simulink model "ex3bSim"  (R2023b)
settings: Solver=VariableStepAuto  StartTime=0.0  StopTime=1000  RelTol=1e-3
values from neighbouring files (symbols this model uses):
  ki = 2    [ex3b.m]
  kp = 2    [ex3b.m]
settings Model: Creator=Bianca  LastModifiedBy=Bianca

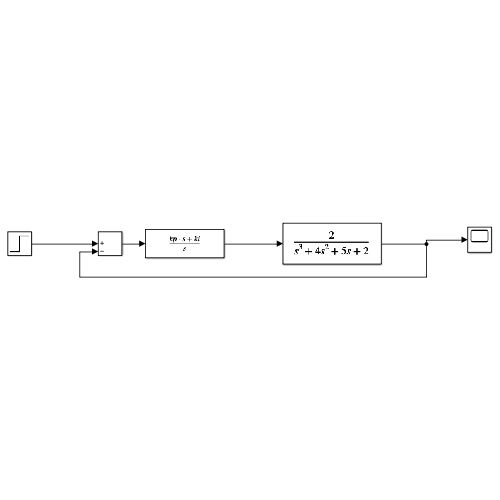
[thumbnail: Simulink's stored preview of the top-level diagram]
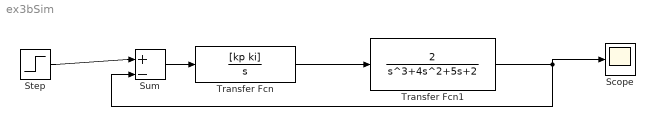
== system ex3bSim ==
  Scope : Scope
  Step : Step  SampleTime=0
  Sum : Sum  Inputs=|+-
  Transfer Fcn : TransferFcn  Numerator=[kp ki]  Denominator=[1 0]
  Transfer Fcn1 : TransferFcn  Numerator=[0 0 0 2]  Denominator=[1 4 5 2]
  wires:
  Step/1 -> Sum/1
  Sum/1 -> Transfer Fcn/1
  Transfer Fcn/1 -> Transfer Fcn1/1
  Transfer Fcn1/1 -> Scope/1, Sum/2
